simulink model "HANcoder_E407_TTA_CombineModel_LR"  (R2023a)
settings: Solver=FixedStepDiscrete  StartTime=0.0  StopTime=1  FixedStep=0.001  RelTol=1e-3
PreLoadFcn:
  | librarySetup
  | eval([bdroot,'_startup']) %Calling [modelName]_startup.m
values from neighbouring files (symbols this model uses):
  ClockOn = Simulink.Parameter    [HANcoder_E407_TTA_Chris_startup.m]    (also in HANcoder_E407_TTA_CombineModel_Membership_2022a_startup.m; HANcoder_E407_TTA_CombineModel_Membership_startup.m; HANcoder_E407_TTA_CombineModel_V2_startup.m; HANcoder_E407_TTA_CombineModel_startup.m)
  controlWidth = Simulink.Parameter    [HANcoder_E407_TTA_CombineModel_Membership_2022a_startup.m]    (also in HANcoder_E407_TTA_CombineModel_Membership_startup.m; HANcoder_E407_TTA_CombineModel_V2_startup.m; HANcoder_E407_TTA_CombineModel_startup.m)
  desiredAngle = Simulink.Parameter    [HANcoder_E407_TTA_CombineModel_Membership_2022a_startup.m]    (also in HANcoder_E407_TTA_CombineModel_Membership_startup.m; HANcoder_E407_TTA_CombineModel_V2_startup.m; HANcoder_E407_TTA_CombineModel_startup.m)
  frequency_IRQ = 1000    [HANcoder_E407_TTA_Chris_startup.m]    (also in HANcoder_E407_TTA_CombineModel_Membership_2022a_startup.m; HANcoder_E407_TTA_CombineModel_Membership_startup.m; HANcoder_E407_TTA_CombineModel_V2_startup.m; HANcoder_E407_TTA_CombineModel_startup.m)
  intVal = Simulink.Parameter    [HANcoder_E407_TTA_CombineModel_Membership_2022a_startup.m]    (also in HANcoder_E407_TTA_CombineModel_Membership_startup.m; HANcoder_E407_TTA_CombineModel_V2_startup.m; HANcoder_E407_TTA_CombineModel_startup.m)
  L0b = 1    [HANcoder_E407_KinematicAngleControl_startup.m]    (also in HANcoder_E407_TTA_CombineModel_Membership_2022a_startup.m; HANcoder_E407_TTA_CombineModel_Membership_startup.m; HANcoder_E407_TTA_CombineModel_V2_startup.m; HANcoder_E407_TTA_CombineModel_startup.m)
  L0F = 3    [HANcoder_E407_KinematicAngleControl_startup.m]    (also in HANcoder_E407_TTA_CombineModel_Membership_2022a_startup.m; HANcoder_E407_TTA_CombineModel_Membership_startup.m; HANcoder_E407_TTA_CombineModel_V2_startup.m; HANcoder_E407_TTA_CombineModel_startup.m)
  L1F = 4    [HANcoder_E407_KinematicAngleControl_startup.m]    (also in HANcoder_E407_TTA_CombineModel_Membership_2022a_startup.m; HANcoder_E407_TTA_CombineModel_Membership_startup.m; HANcoder_E407_TTA_CombineModel_V2_startup.m; HANcoder_E407_TTA_CombineModel_startup.m)
  matrixRows = Simulink.Parameter    [HANcoder_E407_TTA_Chris_startup.m]    (also in HANcoder_E407_TTA_CombineModel_Membership_2022a_startup.m; HANcoder_E407_TTA_CombineModel_Membership_startup.m; HANcoder_E407_TTA_CombineModel_V2_startup.m; HANcoder_E407_TTA_CombineModel_startup.m)
  MMBS1_ID = Simulink.Parameter    [HANcoder_E407_TTA_Chris_startup.m]    (also in HANcoder_E407_TTA_CombineModel_Membership_2022a_startup.m; HANcoder_E407_TTA_CombineModel_Membership_startup.m; HANcoder_E407_TTA_CombineModel_V2_startup.m; HANcoder_E407_TTA_CombineModel_startup.m)
  propVal = Simulink.Parameter    [HANcoder_E407_TTA_CombineModel_Membership_2022a_startup.m]    (also in HANcoder_E407_TTA_CombineModel_Membership_startup.m; HANcoder_E407_TTA_CombineModel_V2_startup.m; HANcoder_E407_TTA_CombineModel_startup.m)
  slotTime = Simulink.Parameter    [HANcoder_E407_TTA_Chris_startup.m]    (also in HANcoder_E407_TTA_CombineModel_Membership_2022a_startup.m; HANcoder_E407_TTA_CombineModel_Membership_startup.m; HANcoder_E407_TTA_CombineModel_V2_startup.m; HANcoder_E407_TTA_CombineModel_startup.m)
  SSTM1_ID = Simulink.Parameter    [HANcoder_E407_TTA_Chris_startup.m]    (also in HANcoder_E407_TTA_CombineModel_Membership_2022a_startup.m; HANcoder_E407_TTA_CombineModel_Membership_startup.m; HANcoder_E407_TTA_CombineModel_V2_startup.m; HANcoder_E407_TTA_CombineModel_startup.m)
  SYNC1_ID = Simulink.Parameter    [HANcoder_E407_TTA_Chris_startup.m]    (also in HANcoder_E407_TTA_CombineModel_Membership_2022a_startup.m; HANcoder_E407_TTA_CombineModel_Membership_startup.m; HANcoder_E407_TTA_CombineModel_V2_startup.m; HANcoder_E407_TTA_CombineModel_startup.m)
  TRCK1_ID1 = Simulink.Parameter    [HANcoder_E407_TTA_Chris_startup.m]    (also in HANcoder_E407_TTA_CombineModel_Membership_2022a_startup.m; HANcoder_E407_TTA_CombineModel_Membership_startup.m; HANcoder_E407_TTA_CombineModel_V2_startup.m; HANcoder_E407_TTA_CombineModel_startup.m)
  TRCK1_ID2 = Simulink.Parameter    [HANcoder_E407_TTA_Chris_startup.m]    (also in HANcoder_E407_TTA_CombineModel_Membership_2022a_startup.m; HANcoder_E407_TTA_CombineModel_Membership_startup.m; HANcoder_E407_TTA_CombineModel_V2_startup.m; HANcoder_E407_TTA_CombineModel_startup.m)
  TRCK1_ID3 = Simulink.Parameter    [HANcoder_E407_TTA_Chris_startup.m]    (also in HANcoder_E407_TTA_CombineModel_Membership_2022a_startup.m; HANcoder_E407_TTA_CombineModel_Membership_startup.m; HANcoder_E407_TTA_CombineModel_V2_startup.m; HANcoder_E407_TTA_CombineModel_startup.m)
  TRLS1_ID4 = Simulink.Parameter    [HANcoder_E407_TTA_Chris_startup.m]    (also in HANcoder_E407_TTA_CombineModel_Membership_2022a_startup.m; HANcoder_E407_TTA_CombineModel_Membership_startup.m; HANcoder_E407_TTA_CombineModel_V2_startup.m; HANcoder_E407_TTA_CombineModel_startup.m)
  TRLS1_ID5 = Simulink.Parameter    [HANcoder_E407_TTA_Chris_startup.m]    (also in HANcoder_E407_TTA_CombineModel_Membership_2022a_startup.m; HANcoder_E407_TTA_CombineModel_Membership_startup.m; HANcoder_E407_TTA_CombineModel_V2_startup.m; HANcoder_E407_TTA_CombineModel_startup.m)
undefined symbols (not defined in the file or in its folder): A2, A3, A4, CON2, CON3, CON4, D10, D4, D5
libraries: HANcoder_STM32_Target x20, hdlsllib x12, dspstat3 x2, simulink x1, slpidlib x1
(part 2 of 3)

== system HANcoder_E407_TTA_CombineModel_LR/HANcoder STM32 Target - E407-STM32 algorithm/Message selector/Subsystem ==
  Trigger : TriggerPort  VariantControl=(inherit)  PortDimensions=1
  Constant : Constant  Value=1.3
  Constant1 : Constant  Value=0
  Control Algorithm : Subsystem
  Data Store Read : DataStoreRead  DataStoreName=requestedAngle  IndexOptions=Index vector (dialog)  Indices=1  OutputSizes=1
  Data Store Read1 : DataStoreRead  DataStoreName=trailerOneAngle  IndexOptions=Index vector (dialog)  Indices=1  OutputSizes=1
  Data Store Read2 : DataStoreRead  DataStoreName=trailerTwoAngle  IndexOptions=Index vector (dialog)  Indices=1  OutputSizes=1
  Data Store Write : DataStoreWrite  DataStoreName=pwmMotor  IndexOptions=Index vector (dialog)  Indices=1  OutputSizes=1
  Data Store Write1 : DataStoreWrite  DataStoreName=cwMotor  IndexOptions=Index vector (dialog)  Indices=1  OutputSizes=1
  Data Store Write8 : DataStoreWrite  DataStoreName=ccwMotor  IndexOptions=Index vector (dialog)  Indices=1  OutputSizes=1
  Kinematic Algorithm : Subsystem
  wires:
  Constant/1 -> Kinematic Algorithm/2(V2)
  Kinematic Algorithm/1(Delta12K) -> Control Algorithm/1(Kinematic output)  "delta12K"
  Data Store Read1/1 -> Kinematic Algorithm/4(YawTrailer1Angle)  "t1Angle"
  Data Store Read/1 -> Kinematic Algorithm/1(DeltaC)  "reqAngle"
  Constant1/1 -> Kinematic Algorithm/3(YawTractorAngle)
  Data Store Read2/1 -> Kinematic Algorithm/5(YawTrailer2Angle)  "t2Angle"
  Control Algorithm/1(Motor speed) -> Data Store Write/1
  Control Algorithm/2(CW direction) -> Data Store Write1/1
  Control Algorithm/3(CCW direction) -> Data Store Write8/1

== system HANcoder_E407_TTA_CombineModel_LR/HANcoder STM32 Target - E407-STM32 algorithm/Message selector/TRCK1_ID2_RX ==
  In1 : Inport
  Enable : EnablePort
  CAN receive1 : Subsystem  Tag=HANcoder_TARGET_STM32_E407  AncestorBlock=HANcoder_STM32_Target/STM32-E407/CAN/CAN/CAN receive  mask(CAN receive){canBus=CAN 1, outputNumber=8, dataType=uint8, byteOrder=off, tsamp=-1}
      mask prompts: canBus "CAN channel"; outputNumber "Output ports"; dataType "Output datatype"; byteOrder "Byte order: Checked = MSB first, unchecked = LSB first."; tsamp "Sample time"
      mask help:
      | Function
      | ==========
      | Receive the newest message from the specified CAN channel.
      |
      | Parameters
      | ==========
      | CAN channel:             The CAN channel to send the message on.
      | Output ports:             The amount of output ports
      | Output datatype:       The datatype of the output ports
      | Byte order:                 Select MSB or LSB first
      | Sample time:              -1 or divisible by base sample time [seconds]
      |
      | Input
      | ==========
      | Port 1:                       CAN ID(uint32) in hexadecimal ie: hex2dec('0a')
      |
      | Output
      | ==========
      | Port 1:                       Checks for new message(int8)
      | Port 2..9                     Message data
      mask init:
      | sfcn_can_receive_mcb(canBus, outputNumber, dataType, byteOrder)
      settings: LibrarySourceBlock=HANcoder_STM32_Target/STM32-E407/CAN/CAN/CAN receive  MoveFcn=drawLogos
      mask Help: web('sfcn_can_receive.html');
      mask TypeOptions canBus: CAN 1 | CAN 2
      mask TypeOptions dataType: int8 | uint8 | int16 | uint16 | int32 | uint32 | boolean
      mask Display:
      | fprintf('Receive on\nCAN %x', canBus);
      | port_label('output', 1, 'new');
      | port_label('input', 1, 'ID');patch([210 216 216],[8 14 2],[1 0 0]);patch([218 218 224],[14 2 8],[0 0 0.35]);
  Terminator{,1..8} (9 alike) : Terminator
  wires:
  CAN receive1/1(Out1) -> Terminator1/1
  CAN receive1/8(Out8) -> Terminator7/1
  CAN receive1/7(Out7) -> Terminator6/1
  CAN receive1/9(Out9) -> Terminator8/1
  CAN receive1/5(Out5) -> Terminator4/1
  CAN receive1/6(Out6) -> Terminator5/1
  CAN receive1/2(Out2) -> Terminator/1
  CAN receive1/4(Out4) -> Terminator3/1
  In1/1 -> CAN receive1/1(In1)
  CAN receive1/3(Out3) -> Terminator2/1

== system HANcoder_E407_TTA_CombineModel_LR/HANcoder STM32 Target - E407-STM32 algorithm/Message selector/TRCK1_ID2_TX ==
  In1 : Inport
  Trigger : TriggerPort  VariantControl=(inherit)  PortDimensions=1
  CAN send1 : Subsystem  Tag=HANcoder_TARGET_STM32_E407  AncestorBlock=HANcoder_STM32_Target/STM32-E407/CAN/CAN/CAN send  mask(CAN send){canBus=CAN 1, frameType=Standard (11 bit), inputNumber=5, dataType=uint8, byteOrder=on, tsamp=-1}
      mask prompts: canBus "CAN channel"; frameType "Identifier type"; inputNumber "Input ports"; dataType "Input datatype"; byteOrder "Byte order: Checked = MSB first, unchecked = LSB first."; tsamp "Sample time"
      mask help:
      | Function
      | ==========
      | Send a message on the CAN channel.
      |
      | Parameters
      | ==========
      | CAN channel:           The CAN channel to send the message on.
      | Identifier type:         normal or extended ID's
      | Input ports:              The amount of input ports
      | Input datatype:        The datatype of the input ports
      | Byte order:               Select MSB or LSB first
      | Sample time:            -1 or divisible by base sample time [seconds]
      |
      | Input
      | ==========
      | Port 1:                   CAN ID(uint32) in hexadecimal ie: hex2dec('0a')
      | Port 2..9                CAN message data
      mask init:
      | sfcn_can_send_mcb(canBus, frameType, inputNumber, dataType, byteOrder)
      settings: LibrarySourceBlock=HANcoder_STM32_Target/STM32-E407/CAN/CAN/CAN send  MoveFcn=drawLogos
      mask Help: web('sfcn_can_send.html');
      mask TypeOptions canBus: CAN 1 | CAN 2
      mask TypeOptions frameType: Standard (11 bit) | Extended (29 bit)
      mask TypeOptions dataType: int8 | uint8 | int16 | uint16 | int32 | uint32 | boolean
      mask Display:
      | fprintf('Send on\nCAN %x', canBus);
      | port_label('input', 1, 'ID');patch([260 266 266],[8 14 2],[1 0 0]);patch([268 268 274],[14 2 8],[0 0 0.35]);
  Data Store Read : DataStoreRead  DataStoreName=potentiometer1  IndexOptions=Index vector (dialog)  Indices=1  OutputSizes=1
  Data Store Read1 : DataStoreRead  DataStoreName=potentiometer2  IndexOptions=Index vector (dialog)  Indices=1  OutputSizes=1
  Data Store Read2 : DataStoreRead  DataStoreName=Local_Ticks  IndexOptions=Index vector (dialog)  Indices=1  OutputSizes=1
  uint16to2uint1 : Subsystem
  uint16to2uint8 : Subsystem
  wires:
  In1/1 -> CAN send1/1(In1)
  uint16to2uint1/1(msb) -> CAN send1/4(In4)
  Data Store Read/1 -> uint16to2uint8/1(input)
  uint16to2uint1/2(lsb) -> CAN send1/5(In5)
  uint16to2uint8/1(msb) -> CAN send1/2(In2)
  Data Store Read1/1 -> uint16to2uint1/1(input)
  uint16to2uint8/2(lsb) -> CAN send1/3(In3)
  Data Store Read2/1 -> CAN send1/6(In6)

== system HANcoder_E407_TTA_CombineModel_LR/HANcoder STM32 Target - E407-STM32 algorithm/Message selector/TRCK1_ID3_TX ==
  In1 : Inport
  Trigger : TriggerPort  VariantControl=(inherit)  PortDimensions=1
  CAN send1 : Subsystem  Tag=HANcoder_TARGET_STM32_E407  AncestorBlock=HANcoder_STM32_Target/STM32-E407/CAN/CAN/CAN send  mask(CAN send){canBus=CAN 1, frameType=Standard (11 bit), inputNumber=5, dataType=uint8, byteOrder=on, tsamp=-1}
      mask prompts: canBus "CAN channel"; frameType "Identifier type"; inputNumber "Input ports"; dataType "Input datatype"; byteOrder "Byte order: Checked = MSB first, unchecked = LSB first."; tsamp "Sample time"
      mask help:
      | Function
      | ==========
      | Send a message on the CAN channel.
      |
      | Parameters
      | ==========
      | CAN channel:           The CAN channel to send the message on.
      | Identifier type:         normal or extended ID's
      | Input ports:              The amount of input ports
      | Input datatype:        The datatype of the input ports
      | Byte order:               Select MSB or LSB first
      | Sample time:            -1 or divisible by base sample time [seconds]
      |
      | Input
      | ==========
      | Port 1:                   CAN ID(uint32) in hexadecimal ie: hex2dec('0a')
      | Port 2..9                CAN message data
      mask init:
      | sfcn_can_send_mcb(canBus, frameType, inputNumber, dataType, byteOrder)
      settings: LibrarySourceBlock=HANcoder_STM32_Target/STM32-E407/CAN/CAN/CAN send  MoveFcn=drawLogos
      mask Help: web('sfcn_can_send.html');
      mask TypeOptions canBus: CAN 1 | CAN 2
      mask TypeOptions frameType: Standard (11 bit) | Extended (29 bit)
      mask TypeOptions dataType: int8 | uint8 | int16 | uint16 | int32 | uint32 | boolean
      mask Display:
      | fprintf('Send on\nCAN %x', canBus);
      | port_label('input', 1, 'ID');patch([200 206 206],[8 14 2],[1 0 0]);patch([208 208 214],[14 2 8],[0 0 0.35]);
  Data Store Read : DataStoreRead  DataStoreName=potentiometer1  IndexOptions=Index vector (dialog)  Indices=1  OutputSizes=1
  Data Store Read1 : DataStoreRead  DataStoreName=potentiometer2  IndexOptions=Index vector (dialog)  Indices=1  OutputSizes=1
  Data Store Read2 : DataStoreRead  DataStoreName=Local_Ticks  IndexOptions=Index vector (dialog)  Indices=1  OutputSizes=1
  uint16to2uint1 : Subsystem
  uint16to2uint8 : Subsystem
  wires:
  In1/1 -> CAN send1/1(In1)
  uint16to2uint1/1(msb) -> CAN send1/4(In4)
  Data Store Read/1 -> uint16to2uint8/1(input)
  uint16to2uint1/2(lsb) -> CAN send1/5(In5)
  uint16to2uint8/1(msb) -> CAN send1/2(In2)
  Data Store Read1/1 -> uint16to2uint1/1(input)
  uint16to2uint8/2(lsb) -> CAN send1/3(In3)
  Data Store Read2/1 -> CAN send1/6(In6)

== system HANcoder_E407_TTA_CombineModel_LR/HANcoder STM32 Target - E407-STM32 algorithm/Message selector/TRCK1_RX ==
  In1 : Inport
  Enable : EnablePort
  CAN receive1 : Subsystem  Tag=HANcoder_TARGET_STM32_E407  AncestorBlock=HANcoder_STM32_Target/STM32-E407/CAN/CAN/CAN receive  mask(CAN receive){canBus=CAN 1, outputNumber=8, dataType=uint8, byteOrder=off, tsamp=-1}
      mask prompts: canBus "CAN channel"; outputNumber "Output ports"; dataType "Output datatype"; byteOrder "Byte order: Checked = MSB first, unchecked = LSB first."; tsamp "Sample time"
      mask help:
      | Function
      | ==========
      | Receive the newest message from the specified CAN channel.
      |
      | Parameters
      | ==========
      | CAN channel:             The CAN channel to send the message on.
      | Output ports:             The amount of output ports
      | Output datatype:       The datatype of the output ports
      | Byte order:                 Select MSB or LSB first
      | Sample time:              -1 or divisible by base sample time [seconds]
      |
      | Input
      | ==========
      | Port 1:                       CAN ID(uint32) in hexadecimal ie: hex2dec('0a')
      |
      | Output
      | ==========
      | Port 1:                       Checks for new message(int8)
      | Port 2..9                     Message data
      mask init:
      | sfcn_can_receive_mcb(canBus, outputNumber, dataType, byteOrder)
      settings: LibrarySourceBlock=HANcoder_STM32_Target/STM32-E407/CAN/CAN/CAN receive  MoveFcn=drawLogos
      mask Help: web('sfcn_can_receive.html');
      mask TypeOptions canBus: CAN 1 | CAN 2
      mask TypeOptions dataType: int8 | uint8 | int16 | uint16 | int32 | uint32 | boolean
      mask Display:
      | fprintf('Receive on\nCAN %x', canBus);
      | port_label('output', 1, 'new');
      | port_label('input', 1, 'ID');patch([210 216 216],[8 14 2],[1 0 0]);patch([218 218 224],[14 2 8],[0 0 0.35]);
  Terminator{,1..8} (9 alike) : Terminator
  wires:
  CAN receive1/1(Out1) -> Terminator1/1
  CAN receive1/8(Out8) -> Terminator7/1
  CAN receive1/7(Out7) -> Terminator6/1
  CAN receive1/9(Out9) -> Terminator8/1
  CAN receive1/5(Out5) -> Terminator4/1
  CAN receive1/6(Out6) -> Terminator5/1
  CAN receive1/2(Out2) -> Terminator/1
  CAN receive1/4(Out4) -> Terminator3/1
  In1/1 -> CAN receive1/1(In1)
  CAN receive1/3(Out3) -> Terminator2/1

== system HANcoder_E407_TTA_CombineModel_LR/HANcoder STM32 Target - E407-STM32 algorithm/Message selector/TRCK1_TX ==
  In1 : Inport
  Trigger : TriggerPort  VariantControl=(inherit)  PortDimensions=1
  CAN send1 : Subsystem  Tag=HANcoder_TARGET_STM32_E407  AncestorBlock=HANcoder_STM32_Target/STM32-E407/CAN/CAN/CAN send  mask(CAN send){canBus=CAN 1, frameType=Standard (11 bit), inputNumber=5, dataType=uint8, byteOrder=on, tsamp=-1}
      mask prompts: canBus "CAN channel"; frameType "Identifier type"; inputNumber "Input ports"; dataType "Input datatype"; byteOrder "Byte order: Checked = MSB first, unchecked = LSB first."; tsamp "Sample time"
      mask help:
      | Function
      | ==========
      | Send a message on the CAN channel.
      |
      | Parameters
      | ==========
      | CAN channel:           The CAN channel to send the message on.
      | Identifier type:         normal or extended ID's
      | Input ports:              The amount of input ports
      | Input datatype:        The datatype of the input ports
      | Byte order:               Select MSB or LSB first
      | Sample time:            -1 or divisible by base sample time [seconds]
      |
      | Input
      | ==========
      | Port 1:                   CAN ID(uint32) in hexadecimal ie: hex2dec('0a')
      | Port 2..9                CAN message data
      mask init:
      | sfcn_can_send_mcb(canBus, frameType, inputNumber, dataType, byteOrder)
      settings: LibrarySourceBlock=HANcoder_STM32_Target/STM32-E407/CAN/CAN/CAN send  MoveFcn=drawLogos
      mask Help: web('sfcn_can_send.html');
      mask TypeOptions canBus: CAN 1 | CAN 2
      mask TypeOptions frameType: Standard (11 bit) | Extended (29 bit)
      mask TypeOptions dataType: int8 | uint8 | int16 | uint16 | int32 | uint32 | boolean
      mask Display:
      | fprintf('Send on\nCAN %x', canBus);
      | port_label('input', 1, 'ID');patch([75 81 81],[8 14 2],[1 0 0]);patch([83 83 89],[14 2 8],[0 0 0.35]);
  Data Store Read : DataStoreRead  DataStoreName=potentiometer1  IndexOptions=Index vector (dialog)  Indices=1  OutputSizes=1
  Data Store Read1 : DataStoreRead  DataStoreName=potentiometer2  IndexOptions=Index vector (dialog)  Indices=1  OutputSizes=1
  Data Store Read2 : DataStoreRead  DataStoreName=Local_Ticks  IndexOptions=Index vector (dialog)  Indices=1  OutputSizes=1
  uint16to2uint1 : Subsystem
  uint16to2uint8 : Subsystem
  wires:
  In1/1 -> CAN send1/1(In1)
  uint16to2uint1/1(msb) -> CAN send1/4(In4)
  Data Store Read/1 -> uint16to2uint8/1(input)
  uint16to2uint1/2(lsb) -> CAN send1/5(In5)
  uint16to2uint8/1(msb) -> CAN send1/2(In2)
  Data Store Read1/1 -> uint16to2uint1/1(input)
  uint16to2uint8/2(lsb) -> CAN send1/3(In3)
  Data Store Read2/1 -> CAN send1/6(In6)

== system HANcoder_E407_TTA_CombineModel_LR/HANcoder STM32 Target - E407-STM32 algorithm/Message selector/TRCK_ID3_RX ==
  In1 : Inport
  Enable : EnablePort
  CAN receive1 : Subsystem  Tag=HANcoder_TARGET_STM32_E407  AncestorBlock=HANcoder_STM32_Target/STM32-E407/CAN/CAN/CAN receive  mask(CAN receive){canBus=CAN 1, outputNumber=8, dataType=uint8, byteOrder=off, tsamp=-1}
      mask prompts: canBus "CAN channel"; outputNumber "Output ports"; dataType "Output datatype"; byteOrder "Byte order: Checked = MSB first, unchecked = LSB first."; tsamp "Sample time"
      mask help:
      | Function
      | ==========
      | Receive the newest message from the specified CAN channel.
      |
      | Parameters
      | ==========
      | CAN channel:             The CAN channel to send the message on.
      | Output ports:             The amount of output ports
      | Output datatype:       The datatype of the output ports
      | Byte order:                 Select MSB or LSB first
      | Sample time:              -1 or divisible by base sample time [seconds]
      |
      | Input
      | ==========
      | Port 1:                       CAN ID(uint32) in hexadecimal ie: hex2dec('0a')
      |
      | Output
      | ==========
      | Port 1:                       Checks for new message(int8)
      | Port 2..9                     Message data
      mask init:
      | sfcn_can_receive_mcb(canBus, outputNumber, dataType, byteOrder)
      settings: LibrarySourceBlock=HANcoder_STM32_Target/STM32-E407/CAN/CAN/CAN receive  MoveFcn=drawLogos
      mask Help: web('sfcn_can_receive.html');
      mask TypeOptions canBus: CAN 1 | CAN 2
      mask TypeOptions dataType: int8 | uint8 | int16 | uint16 | int32 | uint32 | boolean
      mask Display:
      | fprintf('Receive on\nCAN %x', canBus);
      | port_label('output', 1, 'new');
      | port_label('input', 1, 'ID');patch([210 216 216],[8 14 2],[1 0 0]);patch([218 218 224],[14 2 8],[0 0 0.35]);
  Terminator{,1..8} (9 alike) : Terminator
  wires:
  CAN receive1/1(Out1) -> Terminator1/1
  CAN receive1/8(Out8) -> Terminator7/1
  CAN receive1/7(Out7) -> Terminator6/1
  CAN receive1/9(Out9) -> Terminator8/1
  CAN receive1/5(Out5) -> Terminator4/1
  CAN receive1/6(Out6) -> Terminator5/1
  CAN receive1/2(Out2) -> Terminator/1
  CAN receive1/4(Out4) -> Terminator3/1
  In1/1 -> CAN receive1/1(In1)
  CAN receive1/3(Out3) -> Terminator2/1

== system HANcoder_E407_TTA_CombineModel_LR/HANcoder STM32 Target - E407-STM32 algorithm/Message selector/TRLS_ID4_RX ==
  In1 : Inport
  Enable : EnablePort
  2bytes2uint16 : Subsystem
  CAN receive1 : Subsystem  Tag=HANcoder_TARGET_STM32_E407  AncestorBlock=HANcoder_STM32_Target/STM32-E407/CAN/CAN/CAN receive  mask(CAN receive){canBus=CAN 1, outputNumber=8, dataType=uint8, byteOrder=off, tsamp=-1}
      mask prompts: canBus "CAN channel"; outputNumber "Output ports"; dataType "Output datatype"; byteOrder "Byte order: Checked = MSB first, unchecked = LSB first."; tsamp "Sample time"
      mask help:
      | Function
      | ==========
      | Receive the newest message from the specified CAN channel.
      |
      | Parameters
      | ==========
      | CAN channel:             The CAN channel to send the message on.
      | Output ports:             The amount of output ports
      | Output datatype:       The datatype of the output ports
      | Byte order:                 Select MSB or LSB first
      | Sample time:              -1 or divisible by base sample time [seconds]
      |
      | Input
      | ==========
      | Port 1:                       CAN ID(uint32) in hexadecimal ie: hex2dec('0a')
      |
      | Output
      | ==========
      | Port 1:                       Checks for new message(int8)
      | Port 2..9                     Message data
      mask init:
      | sfcn_can_receive_mcb(canBus, outputNumber, dataType, byteOrder)
      settings: LibrarySourceBlock=HANcoder_STM32_Target/STM32-E407/CAN/CAN/CAN receive  MoveFcn=drawLogos
      mask Help: web('sfcn_can_receive.html');
      mask TypeOptions canBus: CAN 1 | CAN 2
      mask TypeOptions dataType: int8 | uint8 | int16 | uint16 | int32 | uint32 | boolean
      mask Display:
      | fprintf('Receive on\nCAN %x', canBus);
      | port_label('output', 1, 'new');
      | port_label('input', 1, 'ID');patch([210 216 216],[8 14 2],[1 0 0]);patch([218 218 224],[14 2 8],[0 0 0.35]);
  Data Store Write : DataStoreWrite  DataStoreName=trailerOneAngle  IndexOptions=Index vector (dialog)  Indices=1  OutputSizes=1
  Gain : Gain  Gain=1/66.66  OutDataTypeStr=uint16  RndMeth=Round
  Terminator{1,3..8} (7 alike) : Terminator
  wires:
  CAN receive1/1(Out1) -> Terminator1/1
  CAN receive1/8(Out8) -> Terminator7/1
  CAN receive1/7(Out7) -> Terminator6/1
  CAN receive1/9(Out9) -> Terminator8/1
  CAN receive1/5(Out5) -> Terminator4/1
  CAN receive1/6(Out6) -> Terminator5/1
  CAN receive1/2(Out2) -> 2bytes2uint16/1(MSB)
  CAN receive1/4(Out4) -> Terminator3/1
  In1/1 -> CAN receive1/1(In1)
  CAN receive1/3(Out3) -> 2bytes2uint16/2(LSB)
  2bytes2uint16/1(uint16Out) -> Gain/1
  Gain/1 -> Data Store Write/1

== system HANcoder_E407_TTA_CombineModel_LR/HANcoder STM32 Target - E407-STM32 algorithm/Message selector/TRLS_ID4_TX ==
  In1 : Inport
  Trigger : TriggerPort  VariantControl=(inherit)  PortDimensions=1
  CAN send1 : Subsystem  Tag=HANcoder_TARGET_STM32_E407  AncestorBlock=HANcoder_STM32_Target/STM32-E407/CAN/CAN/CAN send  mask(CAN send){canBus=CAN 1, frameType=Standard (11 bit), inputNumber=5, dataType=uint8, byteOrder=on, tsamp=-1}
      mask prompts: canBus "CAN channel"; frameType "Identifier type"; inputNumber "Input ports"; dataType "Input datatype"; byteOrder "Byte order: Checked = MSB first, unchecked = LSB first."; tsamp "Sample time"
      mask help:
      | Function
      | ==========
      | Send a message on the CAN channel.
      |
      | Parameters
      | ==========
      | CAN channel:           The CAN channel to send the message on.
      | Identifier type:         normal or extended ID's
      | Input ports:              The amount of input ports
      | Input datatype:        The datatype of the input ports
      | Byte order:               Select MSB or LSB first
      | Sample time:            -1 or divisible by base sample time [seconds]
      |
      | Input
      | ==========
      | Port 1:                   CAN ID(uint32) in hexadecimal ie: hex2dec('0a')
      | Port 2..9                CAN message data
      mask init:
      | sfcn_can_send_mcb(canBus, frameType, inputNumber, dataType, byteOrder)
      settings: LibrarySourceBlock=HANcoder_STM32_Target/STM32-E407/CAN/CAN/CAN send  MoveFcn=drawLogos
      mask Help: web('sfcn_can_send.html');
      mask TypeOptions canBus: CAN 1 | CAN 2
      mask TypeOptions frameType: Standard (11 bit) | Extended (29 bit)
      mask TypeOptions dataType: int8 | uint8 | int16 | uint16 | int32 | uint32 | boolean
      mask Display:
      | fprintf('Send on\nCAN %x', canBus);
      | port_label('input', 1, 'ID');patch([175 181 181],[8 14 2],[1 0 0]);patch([183 183 189],[14 2 8],[0 0 0.35]);
  Data Store Read : DataStoreRead  DataStoreName=potentiometer1  IndexOptions=Index vector (dialog)  Indices=1  OutputSizes=1
  Data Store Read1 : DataStoreRead  DataStoreName=potentiometer2  IndexOptions=Index vector (dialog)  Indices=1  OutputSizes=1
  Data Store Read2 : DataStoreRead  DataStoreName=Local_Ticks  IndexOptions=Index vector (dialog)  Indices=1  OutputSizes=1
  uint16to2uint1 : Subsystem
  uint16to2uint8 : Subsystem
  wires:
  In1/1 -> CAN send1/1(In1)
  Data Store Read/1 -> uint16to2uint8/1(input)
  uint16to2uint8/1(msb) -> CAN send1/2(In2)
  uint16to2uint8/2(lsb) -> CAN send1/3(In3)
  Data Store Read1/1 -> uint16to2uint1/1(input)
  uint16to2uint1/1(msb) -> CAN send1/4(In4)
  uint16to2uint1/2(lsb) -> CAN send1/5(In5)
  Data Store Read2/1 -> CAN send1/6(In6)

== system HANcoder_E407_TTA_CombineModel_LR/HANcoder STM32 Target - E407-STM32 algorithm/Message selector/TRLS_ID5_RX ==
  In1 : Inport
  Enable : EnablePort
  2bytes2uint16 : Subsystem
  CAN receive1 : Subsystem  Tag=HANcoder_TARGET_STM32_E407  AncestorBlock=HANcoder_STM32_Target/STM32-E407/CAN/CAN/CAN receive  mask(CAN receive){canBus=CAN 1, outputNumber=8, dataType=uint8, byteOrder=off, tsamp=-1}
      mask prompts: canBus "CAN channel"; outputNumber "Output ports"; dataType "Output datatype"; byteOrder "Byte order: Checked = MSB first, unchecked = LSB first."; tsamp "Sample time"
      mask help:
      | Function
      | ==========
      | Receive the newest message from the specified CAN channel.
      |
      | Parameters
      | ==========
      | CAN channel:             The CAN channel to send the message on.
      | Output ports:             The amount of output ports
      | Output datatype:       The datatype of the output ports
      | Byte order:                 Select MSB or LSB first
      | Sample time:              -1 or divisible by base sample time [seconds]
      |
      | Input
      | ==========
      | Port 1:                       CAN ID(uint32) in hexadecimal ie: hex2dec('0a')
      |
      | Output
      | ==========
      | Port 1:                       Checks for new message(int8)
      | Port 2..9                     Message data
      mask init:
      | sfcn_can_receive_mcb(canBus, outputNumber, dataType, byteOrder)
      settings: LibrarySourceBlock=HANcoder_STM32_Target/STM32-E407/CAN/CAN/CAN receive  MoveFcn=drawLogos
      mask Help: web('sfcn_can_receive.html');
      mask TypeOptions canBus: CAN 1 | CAN 2
      mask TypeOptions dataType: int8 | uint8 | int16 | uint16 | int32 | uint32 | boolean
      mask Display:
      | fprintf('Receive on\nCAN %x', canBus);
      | port_label('output', 1, 'new');
      | port_label('input', 1, 'ID');patch([210 216 216],[8 14 2],[1 0 0]);patch([218 218 224],[14 2 8],[0 0 0.35]);
  Data Store Write1 : DataStoreWrite  DataStoreName=trailerTwoAngle  IndexOptions=Index vector (dialog)  Indices=1  OutputSizes=1
  Gain : Gain  Gain=1/66.66  OutDataTypeStr=uint16  RndMeth=Round
  Terminator{1,3..8} (7 alike) : Terminator
  wires:
  CAN receive1/1(Out1) -> Terminator1/1
  CAN receive1/8(Out8) -> Terminator7/1
  CAN receive1/7(Out7) -> Terminator6/1
  CAN receive1/9(Out9) -> Terminator8/1
  CAN receive1/5(Out5) -> Terminator4/1
  CAN receive1/6(Out6) -> Terminator5/1
  CAN receive1/2(Out2) -> 2bytes2uint16/1(MSB)
  CAN receive1/4(Out4) -> Terminator3/1
  In1/1 -> CAN receive1/1(In1)
  CAN receive1/3(Out3) -> 2bytes2uint16/2(LSB)
  2bytes2uint16/1(uint16Out) -> Gain/1
  Gain/1 -> Data Store Write1/1

== system HANcoder_E407_TTA_CombineModel_LR/HANcoder STM32 Target - E407-STM32 algorithm/Message selector/TRLS_ID5_TX ==
  In1 : Inport
  Trigger : TriggerPort  VariantControl=(inherit)  PortDimensions=1
  CAN send1 : Subsystem  Tag=HANcoder_TARGET_STM32_E407  AncestorBlock=HANcoder_STM32_Target/STM32-E407/CAN/CAN/CAN send  mask(CAN send){canBus=CAN 1, frameType=Standard (11 bit), inputNumber=5, dataType=uint8, byteOrder=on, tsamp=-1}
      mask prompts: canBus "CAN channel"; frameType "Identifier type"; inputNumber "Input ports"; dataType "Input datatype"; byteOrder "Byte order: Checked = MSB first, unchecked = LSB first."; tsamp "Sample time"
      mask help:
      | Function
      | ==========
      | Send a message on the CAN channel.
      |
      | Parameters
      | ==========
      | CAN channel:           The CAN channel to send the message on.
      | Identifier type:         normal or extended ID's
      | Input ports:              The amount of input ports
      | Input datatype:        The datatype of the input ports
      | Byte order:               Select MSB or LSB first
      | Sample time:            -1 or divisible by base sample time [seconds]
      |
      | Input
      | ==========
      | Port 1:                   CAN ID(uint32) in hexadecimal ie: hex2dec('0a')
      | Port 2..9                CAN message data
      mask init:
      | sfcn_can_send_mcb(canBus, frameType, inputNumber, dataType, byteOrder)
      settings: LibrarySourceBlock=HANcoder_STM32_Target/STM32-E407/CAN/CAN/CAN send  MoveFcn=drawLogos
      mask Help: web('sfcn_can_send.html');
      mask TypeOptions canBus: CAN 1 | CAN 2
      mask TypeOptions frameType: Standard (11 bit) | Extended (29 bit)
      mask TypeOptions dataType: int8 | uint8 | int16 | uint16 | int32 | uint32 | boolean
      mask Display:
      | fprintf('Send on\nCAN %x', canBus);
      | port_label('input', 1, 'ID');patch([200 206 206],[8 14 2],[1 0 0]);patch([208 208 214],[14 2 8],[0 0 0.35]);
  Data Store Read1 : DataStoreRead  DataStoreName=potentiometer1  IndexOptions=Index vector (dialog)  Indices=1  OutputSizes=1
  Data Store Read2 : DataStoreRead  DataStoreName=potentiometer2  IndexOptions=Index vector (dialog)  Indices=1  OutputSizes=1
  Data Store Read3 : DataStoreRead  DataStoreName=Local_Ticks  IndexOptions=Index vector (dialog)  Indices=1  OutputSizes=1
  uint16to2uint1 : Subsystem
  uint16to2uint2 : Subsystem
  wires:
  In1/1 -> CAN send1/1(In1)
  Data Store Read1/1 -> uint16to2uint2/1(input)
  Data Store Read2/1 -> uint16to2uint1/1(input)
  uint16to2uint2/2(lsb) -> CAN send1/3(In3)
  uint16to2uint2/1(msb) -> CAN send1/2(In2)
  uint16to2uint1/1(msb) -> CAN send1/4(In4)
  uint16to2uint1/2(lsb) -> CAN send1/5(In5)
  Data Store Read3/1 -> CAN send1/6(In6)

== system HANcoder_E407_TTA_CombineModel_LR/HANcoder STM32 Target - E407-STM32 algorithm/Role assignment/Subsystem ==
  Trigger : TriggerPort  VariantControl=(inherit)  PortDimensions=1
  Constant1 : Constant  Value=0  OutDataTypeStr=uint8
  Constant3 : Constant  Value=slotTime  OutDataTypeStr=uint8
  Data Store Write : DataStoreWrite  DataStoreName=SlotTime  IndexOptions=Index vector (dialog)  Indices=1  OutputSizes=1
  Data Store Write1 : DataStoreWrite  DataStoreName=Local_Ticks  IndexOptions=Index vector (dialog)  Indices=1  OutputSizes=1
  wires:
  Constant3/1 -> Data Store Write/1
  Constant1/1 -> Data Store Write1/1

== system HANcoder_E407_TTA_CombineModel_LR/HANcoder STM32 Target - E407-STM32 algorithm/Role assignment/Subsystem2 ==
  Enable : EnablePort
  CAN receive1 : Subsystem  Tag=HANcoder_TARGET_STM32_E407  AncestorBlock=HANcoder_STM32_Target/STM32-E407/CAN/CAN/CAN receive  mask(CAN receive){canBus=CAN 1, outputNumber=8, dataType=uint8, byteOrder=off, tsamp=-1}
      mask prompts: canBus "CAN channel"; outputNumber "Output ports"; dataType "Output datatype"; byteOrder "Byte order: Checked = MSB first, unchecked = LSB first."; tsamp "Sample time"
      mask help:
      | Function
      | ==========
      | Receive the newest message from the specified CAN channel.
      |
      | Parameters
      | ==========
      | CAN channel:             The CAN channel to send the message on.
      | Output ports:             The amount of output ports
      | Output datatype:       The datatype of the output ports
      | Byte order:                 Select MSB or LSB first
      | Sample time:              -1 or divisible by base sample time [seconds]
      |
      | Input
      | ==========
      | Port 1:                       CAN ID(uint32) in hexadecimal ie: hex2dec('0a')
      |
      | Output
      | ==========
      | Port 1:                       Checks for new message(int8)
      | Port 2..9                     Message data
      mask init:
      | sfcn_can_receive_mcb(canBus, outputNumber, dataType, byteOrder)
      settings: LibrarySourceBlock=HANcoder_STM32_Target/STM32-E407/CAN/CAN/CAN receive  MoveFcn=drawLogos
      mask Help: web('sfcn_can_receive.html');
      mask TypeOptions canBus: CAN 1 | CAN 2
      mask TypeOptions dataType: int8 | uint8 | int16 | uint16 | int32 | uint32 | boolean
      mask Display:
      | fprintf('Receive on\nCAN %x', canBus);
      | port_label('output', 1, 'new');
      | port_label('input', 1, 'ID');patch([210 216 216],[8 14 2],[1 0 0]);patch([218 218 224],[14 2 8],[0 0 0.35]);
  Constant10 : Constant  Value=SYNC1_ID  OutDataTypeStr=uint32
  Subsystem1 : Subsystem
  Terminator{1,3..8} (7 alike) : Terminator
  wires:
  CAN receive1/4(Out4) -> Terminator3/1
  CAN receive1/5(Out5) -> Terminator4/1
  CAN receive1/3(Out3) -> Terminator1/1
  CAN receive1/1(Out1) -> Subsystem1/Trigger
  CAN receive1/8(Out8) -> Terminator7/1
  CAN receive1/6(Out6) -> Terminator5/1
  CAN receive1/7(Out7) -> Terminator6/1
  CAN receive1/9(Out9) -> Terminator8/1
  CAN receive1/2(Out2) -> Subsystem1/1(dataArx)
  Constant10/1 -> CAN receive1/1(In1)

== system HANcoder_E407_TTA_CombineModel_LR/HANcoder STM32 Target - E407-STM32 algorithm/Message selector/MMBS1_RX/CAN receive1 ==
  In1 : Inport
  Enabled Subsystem : Subsystem  TreatAsAtomicUnit=on
  S-Function : M-S-Function  FunctionName=sfcn_can_receive  Parameters=tsamp, canBus, outputNumber, dataType, byteOrder
  Out1 : Outport
  Out2 : Outport  Port=2
  Out3 : Outport  Port=3
  Out4 : Outport  Port=4
  Out5 : Outport  Port=5
  Out6 : Outport  Port=6
  Out7 : Outport  Port=7
  Out8 : Outport  Port=8
  Out9 : Outport  Port=9
  wires:
  S-Function/9 -> Enabled Subsystem/8(In8)
  S-Function/4 -> Enabled Subsystem/3(In3)
  S-Function/5 -> Enabled Subsystem/4(In4)
  S-Function/8 -> Enabled Subsystem/7(In7)
  S-Function/7 -> Enabled Subsystem/6(In6)
  S-Function/6 -> Enabled Subsystem/5(In5)
  Enabled Subsystem/8(Out8) -> Out9/1
  Enabled Subsystem/7(Out7) -> Out8/1
  Enabled Subsystem/6(Out6) -> Out7/1
  Enabled Subsystem/5(Out5) -> Out6/1
  Enabled Subsystem/4(Out4) -> Out5/1
  Enabled Subsystem/3(Out3) -> Out4/1
  Enabled Subsystem/2(Out2) -> Out3/1
  Enabled Subsystem/1(Out1) -> Out2/1
  S-Function/3 -> Enabled Subsystem/2(In2)
  S-Function/2 -> Enabled Subsystem/1(In1)
  S-Function/1 -> Out1/1, Enabled Subsystem/Enable
  In1/1 -> S-Function/1

== system HANcoder_E407_TTA_CombineModel_LR/HANcoder STM32 Target - E407-STM32 algorithm/Message selector/MMBS1_TX/CAN send1 ==
  In1 : Inport
  In2 : Inport  Port=2
  Gnd{3..9} (7 alike) : Ground
  S-Function : M-S-Function  FunctionName=sfcn_can_send  Parameters=tsamp, canBus, frameType, inputNumber, dataType, byteOrder
  wires:
  In1/1 -> S-Function/1
  In2/1 -> S-Function/2
  Gnd3/1 -> S-Function/3
  Gnd4/1 -> S-Function/4
  Gnd5/1 -> S-Function/5
  Gnd6/1 -> S-Function/6
  Gnd7/1 -> S-Function/7
  Gnd8/1 -> S-Function/8
  Gnd9/1 -> S-Function/9

== system HANcoder_E407_TTA_CombineModel_LR/HANcoder STM32 Target - E407-STM32 algorithm/Message selector/SSTM1_RX/CAN receive1 ==
  In1 : Inport
  Enabled Subsystem : Subsystem  TreatAsAtomicUnit=on
  S-Function : M-S-Function  FunctionName=sfcn_can_receive  Parameters=tsamp, canBus, outputNumber, dataType, byteOrder
  Out1 : Outport
  Out2 : Outport  Port=2
  Out3 : Outport  Port=3
  Out4 : Outport  Port=4
  Out5 : Outport  Port=5
  Out6 : Outport  Port=6
  Out7 : Outport  Port=7
  Out8 : Outport  Port=8
  Out9 : Outport  Port=9
  wires:
  S-Function/9 -> Enabled Subsystem/8(In8)
  S-Function/4 -> Enabled Subsystem/3(In3)
  S-Function/5 -> Enabled Subsystem/4(In4)
  S-Function/8 -> Enabled Subsystem/7(In7)
  S-Function/7 -> Enabled Subsystem/6(In6)
  S-Function/6 -> Enabled Subsystem/5(In5)
  Enabled Subsystem/8(Out8) -> Out9/1
  Enabled Subsystem/7(Out7) -> Out8/1
  Enabled Subsystem/6(Out6) -> Out7/1
  Enabled Subsystem/5(Out5) -> Out6/1
  Enabled Subsystem/4(Out4) -> Out5/1
  Enabled Subsystem/3(Out3) -> Out4/1
  Enabled Subsystem/2(Out2) -> Out3/1
  Enabled Subsystem/1(Out1) -> Out2/1
  S-Function/3 -> Enabled Subsystem/2(In2)
  S-Function/2 -> Enabled Subsystem/1(In1)
  S-Function/1 -> Out1/1, Enabled Subsystem/Enable
  In1/1 -> S-Function/1

== system HANcoder_E407_TTA_CombineModel_LR/HANcoder STM32 Target - E407-STM32 algorithm/Message selector/SSTM1_TX/CAN send1 ==
  In1 : Inport
  In2 : Inport  Port=2
  Gnd{3..9} (7 alike) : Ground
  S-Function : M-S-Function  FunctionName=sfcn_can_send  Parameters=tsamp, canBus, frameType, inputNumber, dataType, byteOrder
  wires:
  In1/1 -> S-Function/1
  In2/1 -> S-Function/2
  Gnd3/1 -> S-Function/3
  Gnd4/1 -> S-Function/4
  Gnd5/1 -> S-Function/5
  Gnd6/1 -> S-Function/6
  Gnd7/1 -> S-Function/7
  Gnd8/1 -> S-Function/8
  Gnd9/1 -> S-Function/9

== system HANcoder_E407_TTA_CombineModel_LR/HANcoder STM32 Target - E407-STM32 algorithm/Message selector/SYNC1_RX/CAN receive1 ==
  In1 : Inport
  Enabled Subsystem : Subsystem  TreatAsAtomicUnit=on
  S-Function : M-S-Function  FunctionName=sfcn_can_receive  Parameters=tsamp, canBus, outputNumber, dataType, byteOrder
  Out1 : Outport
  Out2 : Outport  Port=2
  Out3 : Outport  Port=3
  Out4 : Outport  Port=4
  Out5 : Outport  Port=5
  Out6 : Outport  Port=6
  Out7 : Outport  Port=7
  Out8 : Outport  Port=8
  Out9 : Outport  Port=9
  wires:
  S-Function/9 -> Enabled Subsystem/8(In8)
  S-Function/4 -> Enabled Subsystem/3(In3)
  S-Function/5 -> Enabled Subsystem/4(In4)
  S-Function/8 -> Enabled Subsystem/7(In7)
  S-Function/7 -> Enabled Subsystem/6(In6)
  S-Function/6 -> Enabled Subsystem/5(In5)
  Enabled Subsystem/8(Out8) -> Out9/1
  Enabled Subsystem/7(Out7) -> Out8/1
  Enabled Subsystem/6(Out6) -> Out7/1
  Enabled Subsystem/5(Out5) -> Out6/1
  Enabled Subsystem/4(Out4) -> Out5/1
  Enabled Subsystem/3(Out3) -> Out4/1
  Enabled Subsystem/2(Out2) -> Out3/1
  Enabled Subsystem/1(Out1) -> Out2/1
  S-Function/3 -> Enabled Subsystem/2(In2)
  S-Function/2 -> Enabled Subsystem/1(In1)
  S-Function/1 -> Out1/1, Enabled Subsystem/Enable
  In1/1 -> S-Function/1

== system HANcoder_E407_TTA_CombineModel_LR/HANcoder STM32 Target - E407-STM32 algorithm/Message selector/SYNC1_RX/Subsystem ==
  dataArx : Inport
  Trigger : TriggerPort  VariantControl=(inherit)  PortDimensions=1
  Constant : Constant  Value=2  OutDataTypeStr=uint8
  Constant1 : Constant  OutDataTypeStr=uint8
  Data Store Write : DataStoreWrite  DataStoreName=SlotTime  IndexOptions=Index vector (dialog)  Indices=1  OutputSizes=1
  Data Store Write1 : DataStoreWrite  DataStoreName=Local_Ticks  IndexOptions=Index vector (dialog)  Indices=1  OutputSizes=1
  Data Store Write2 : DataStoreWrite  DataStoreName=slot  IndexOptions=Index vector (dialog)  Indices=1  OutputSizes=1
  wires:
  dataArx/1 -> Data Store Write/1
  Constant/1 -> Data Store Write1/1
  Constant1/1 -> Data Store Write2/1

== system HANcoder_E407_TTA_CombineModel_LR/HANcoder STM32 Target - E407-STM32 algorithm/Message selector/SYNC1_TX/CAN send1 ==
  In1 : Inport
  In2 : Inport  Port=2
  In3 : Inport  Port=3
  In4 : Inport  Port=4
  In5 : Inport  Port=5
  In6 : Inport  Port=6
  In7 : Inport  Port=7
  In8 : Inport  Port=8
  In9 : Inport  Port=9
  S-Function : M-S-Function  FunctionName=sfcn_can_send  Parameters=tsamp, canBus, frameType, inputNumber, dataType, byteOrder
  wires:
  In1/1 -> S-Function/1
  In2/1 -> S-Function/2
  In3/1 -> S-Function/3
  In4/1 -> S-Function/4
  In5/1 -> S-Function/5
  In6/1 -> S-Function/6
  In7/1 -> S-Function/7
  In8/1 -> S-Function/8
  In9/1 -> S-Function/9

== system HANcoder_E407_TTA_CombineModel_LR/HANcoder STM32 Target - E407-STM32 algorithm/Message selector/Slot 5 execution/Inputs ==
  note: The inputs and outputs are kept in a separate subsystem, this way the algorithm can easily be transferred to different hardware
  note: The gains here are to determine the angles from 0 - 60
  Cast{,1..3} (4 alike) : DataTypeConversion  SaturateOnIntegerOverflow=off  RndMeth=Floor
  Constant2 : Constant  Value=desiredAngle
  Data Store Write : DataStoreWrite  DataStoreName=encoderPosition  IndexOptions=Index vector (dialog)  Indices=1  OutputSizes=1
  Data Store Write1 : DataStoreWrite  DataStoreName=potentiometer1  IndexOptions=Index vector (dialog)  Indices=1  OutputSizes=1
  Data Store Write2 : DataStoreWrite  DataStoreName=requestedAngle  IndexOptions=Index vector (dialog)  Indices=1  OutputSizes=1
  Data Store Write3 : DataStoreWrite  DataStoreName=potentiometer2  IndexOptions=Index vector (dialog)  Indices=1  OutputSizes=1
  Gain : Gain  Gain=1/66.66  OutDataTypeStr=double  RndMeth=Round
  Moving Average : dspstat3/Moving Average  Method=Sliding window  ForgettingFactorPort=off  SpecifyWindowLength=on  WindowLength=60  OverlapLength=59  AllowArbitraryInputLength=off  ForgettingFactor=0.9  SimulateUsing=Code generation
  Moving Average1 : dspstat3/Moving Average  Method=Sliding window  ForgettingFactorPort=off  SpecifyWindowLength=on  WindowLength=60  OverlapLength=59  AllowArbitraryInputLength=off  ForgettingFactor=0.9  SimulateUsing=Code generation
  Quadrature Encoder Get : Subsystem  Tag=HANcoder_TARGET_STM32_E407  AncestorBlock=HANcoder_STM32_Target/STM32-E407/Timer Inputs/Quadrature Encoder Get  mask(Quadrature Encoder Inputs){moduleID=TIM3: CON4 - D12 & D11 (5V Tolerant), config=Floating, counterReset=off, tsamp=-1}
      mask prompts: moduleID "Quad encoder module"; config "Configuration"; counterReset "Show counter reset input"; tsamp "Sample time"
      mask help:
      | Function
      | ========
      | Reads the counter of the quadrature encoder module.
      |
      | Parameters
      | ==========
      | Quadrature encoder module:
      |   Selects the quadrature encoder module. The channel A and B signals of the
      |   encoder should be connected to the 2 input pins that belong to the module.
      |
      | Configuration:
      |   Determines if the input is floating or is connected to an internal
      |   pull-up or pull-down resistor.
      |
      | Show counter reset input:
      |   Configures if the input port for the counter reset should be shown.
      |
      |
      | Outport
      | ==========
      | 32-bit signed counter. The counter starts at zero and counts up or down
      | depending on the direction of the motor.
      mask init:
      | moduleIDInfoStr = sfcn_quad_encoder_get_mcb(2,moduleID, counterReset, config);
      settings: LibrarySourceBlock=HANcoder_STM32_Target/STM32-E407/Timer Inputs/Quadrature Encoder Get  CopyFcn=sfcn_quad_encoder_get_chk();  MoveFcn=drawLogos
      mask Help: web('sfcn_quad_encoder_get.html');
      mask TypeOptions moduleID: TIM1: CON PE - 12 & 14 (5V Tolerant) | TIM3: CON4 - D12 & D11 (5V Tolerant) | TIM4: CON PD - 15 & 16 (5V Tolerant) | TIM8: UEXT - 3 & 4 (5V Tolerant)
      mask Callback moduleID: sfcn_quad_encoder_get_chk();
      mask TypeOptions config: Floating | Pullup | Pulldown
      mask Display: fprintf('Quad Encoder Get\n%s', moduleIDInfoStr);patch([135 141 141],[8 14 2],[1 0 0]);patch([143 143 149],[14 2 8],[0 0 0.35]);
  Trailer1 Angle : HANcoder_STM32_Target/STM32-E407/Analog Inputs/Analog Input  Tag=HANcoder_TARGET_STM32_E407  pinID=CON2 - A2  tsamp=-1  filtered=off
      settings: SourceProductName=HANcoder STM32 Target
  Trailer2 Angle : HANcoder_STM32_Target/STM32-E407/Analog Inputs/Analog Input  Tag=HANcoder_TARGET_STM32_E407  pinID=CON2 - A3  tsamp=-1  filtered=off
      settings: SourceProductName=HANcoder STM32 Target
  wires:
  Constant2/1 -> Gain/1
  Gain/1 -> Data Store Write2/1
  Quadrature Encoder Get/1(Out1) -> Data Store Write/1
  Trailer1 Angle/1 -> Cast/1  "analogPot1"
  Trailer2 Angle/1 -> Cast3/1  "analogPot2"
  Moving Average/1 -> Cast1/1
  Moving Average1/1 -> Cast2/1
  Cast/1 -> Moving Average/1
  Cast1/1 -> Data Store Write1/1  "pot1"
  Cast2/1 -> Data Store Write3/1  "pot2"
  Cast3/1 -> Moving Average1/1

== system HANcoder_E407_TTA_CombineModel_LR/HANcoder STM32 Target - E407-STM32 algorithm/Message selector/Slot 5 execution/Outputs ==
  note: The inputs and outputs are kept in a separate subsystem, this way the algorithm can easily be transferred to different hardware
  PWM mospeed : Inport
  CW signal : Inport  Port=2
  CCW signal : Inport  Port=3
  Digital Output : HANcoder_STM32_Target/STM32-E407/Digital Outputs/Digital Output  Tag=HANcoder_TARGET_STM32_E407  pinID=CON3 - D4  config=Push pull  tsamp=-1
      settings: SourceProductName=HANcoder STM32 Target
  Digital Output1 : HANcoder_STM32_Target/STM32-E407/Digital Outputs/Digital Output  Tag=HANcoder_TARGET_STM32_E407  pinID=CON3 - D5  config=Push pull  tsamp=-1
      settings: SourceProductName=HANcoder STM32 Target
  PWM Duty Cycle : HANcoder_STM32_Target/STM32-E407/PWM Outputs/PWM Duty Cycle  Tag=HANcoder_TARGET_STM32_E407  pinID=CON2 - A4  tsamp=-1
      settings: SourceProductName=HANcoder STM32 Target
  PWM Init : Subsystem  Tag=HANcoder_TARGET_STM32_E407  AncestorBlock=HANcoder_STM32_Target/STM32-E407/PWM Outputs/PWM Init  mask(Pulse Width Modulation Initialization){moduleID=TIM14: A4 & n/a & n/a & n/a, frequency=10253, alignment=Edge aligned, enableIRQoutput=off, ch1On=on, ch1Pol=Active high, ch1Inv=off, ch2On=on, ch2Pol=Active high, ch2Inv=off, ch3On=off, ch3Pol=Active high, ch3Inv=off, ch4On=off, ch4Pol=Active high, ch4Inv=off}
      mask prompts: moduleID "PWM module"; frequency "Signal frequency [Hz]"; alignment "Signal alignment"; enableIRQoutput "Enable IRQ output"; ch1On "Generate PWM signal on channel 1"; ch1Pol "Select signal polarity"; ch1Inv "Enable inverted signal on additional output pin"; ch2On "Generate PWM signal on channel 2"; ch2Pol "Select signal polarity"; ch2Inv "Enable inverted signal on additional output pin"; ch3On "Generate PWM signal on channel 3"; ch3Pol "Select signal polarity"; ch3Inv "Enable inverted signal on additional output pin"; ch4On "Generate PWM signal on channel 4"; ch4Pol "Select signal polarity"; ch4Inv "Enable inverted signal on additional output pin"
      mask help:
      | Function
      | ========
      | A 'PWM Init' block configures one of the STM32 timer modules for PWM
      | functionality, allowing a PWM signal to be generated on up to 4 timer
      | channels and their associated output pins.
      |
      | Parameters
      | ==========
      | General - PWM module:
      |   Select the PWM module to use. The name in the combo box contains
      |   information about which pins on the target belong to this timer module.
      |   Also the first pin corresponds with the first channel and so on:
      |   TIMx: Ch1 & Ch2 & Ch3...
      |
      | General - Signal frequency:
      |   Determines the signal frequency in Hz. If you click 'Apply' after entering
      |   the desired frequency it will automatically be adjusted to the closest
      |   supported value.
      |
      | General - Signal Aligment:
      |   Determines the aligment of the signal. It can either be edge aligned or
      |   center aligned.
      |
      | General - Enable IRQ output
      |   Controls whether or not the IRQ output is available.
      |
      | Channel x - Generate PWM signal on channel x:
      |   Enable to configure the channel for PWM functionality so that the PWM signal
      |   is outputted on the channel's associated microcontroller pin.
      |
      | Channel x - Signal polarity:
      |   Selects the polarity of the signal.
      |
      | Channel x - Enable inverted signal on additional output pin:
      |   When enabled, a second PWM signal will be generated on an additional
      |   microcontroller pin where the signal is an exact inversion of the first signal.
      mask init:
      | moduleIDInfoStr = sfcn_pwmout_init_mcb(2, moduleID, frequency, alignment, enableIRQoutput, ch1On, ch2On, ch3On, ch4On, ch1Pol, ch2Pol, ch3Pol, ch4Pol, ch1Inv, ch2Inv, ch3Inv, ch4Inv);
      settings: LibrarySourceBlock=HANcoder_STM32_Target/STM32-E407/PWM Outputs/PWM Init  CopyFcn=sfcn_pwmout_init_chk();  MoveFcn=drawLogos
      mask Help: web('sfcn_pwmout_init.html');
      mask TypeOptions moduleID: TIM1:   PE12 & PE14 & PE16 & PE17 + N-channels PE11 & PE13 & PE15 | TIM2:   D13 & n/a & n/a & n/a | TIM3:   D12 & D11 & n/a & n/a | TIM4:   PD15 & PD16 &n/a & n/a | TIM8:   UEXT3 & UEXT4 & n/a & n/a | TIM9:   D4 & D5 & n/a & n/a | TIM10: A1 & n/a & n/a & n/a | TIM11: A2 & n/a & n/a & n/a | TIM13: A3 & n/a & n/a & n/a | TIM14: A4 & n/a & n/a & n/a
      mask Callback moduleID: sfcn_pwmout_init_chk();
      mask TypeOptions alignment: Edge aligned | Center aligned
      mask TypeOptions ch1Pol: Active high | Active low
      mask TypeOptions ch2Pol: Active high | Active low
      mask TypeOptions ch3Pol: Active high | Active low
      mask TypeOptions ch4Pol: Active high | Active low
      mask Display: fprintf('PWM Init\n%s', moduleIDInfoStr);patch([195 201 201],[8 14 2],[1 0 0]);patch([203 203 209],[14 2 8],[0 0 0.35]);
  wires:
  CCW signal/1 -> Digital Output1/1
  CW signal/1 -> Digital Output/1
  PWM mospeed/1 -> PWM Duty Cycle/1
